simulink model "spi"  (Simulink 7.3)
settings: Solver=ode45  StartTime=0.0  StopTime=10.0  RelTol=1e-3
libraries: powerlib x11
settings Model: Creator=vlc  LastModifiedBy=vlc

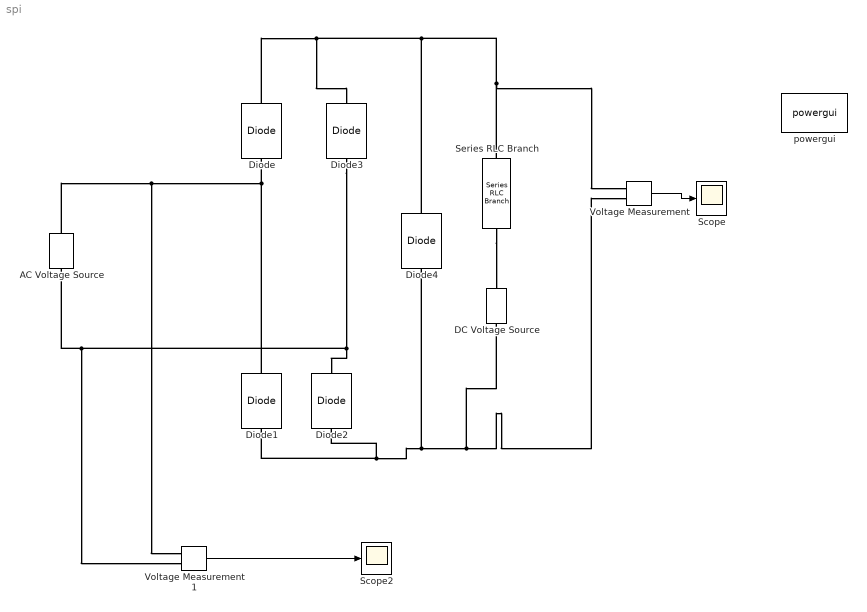
== system spi ==
  AC Voltage Source : powerlib/Electrical Sources/AC Voltage Source  DialogController=POWERSYS.PowerSysDialog  SystemSampleTime=-1  Amplitude=230  Phase=0  Frequency=50  SampleTime=0  Measurements=Voltage
  DC Voltage Source : powerlib/Electrical Sources/DC Voltage Source  DialogController=POWERSYS.PowerSysDialog  SystemSampleTime=-1  Amplitude=60  Measurements=None
  Diode : powerlib/Power Electronics/Diode  DialogController=POWERSYS.PowerSysDialog  SystemSampleTime=-1  Ron=.001  Lon=0  Vf=0.8  IC=0  UseSnubber=off  Rs=500  Cs=.0001  Measurements=off
  Diode1 : powerlib/Power Electronics/Diode  DialogController=POWERSYS.PowerSysDialog  SystemSampleTime=-1  Ron=0.001  Lon=0  Vf=0.8  IC=0  UseSnubber=off  Rs=500  Cs=.0001  Measurements=off
  Diode2 : powerlib/Power Electronics/Diode  DialogController=POWERSYS.PowerSysDialog  SystemSampleTime=-1  Ron=0.001  Lon=0  Vf=0.8  IC=0  UseSnubber=off  Rs=500  Cs=.0001  Measurements=off
  Diode3 : powerlib/Power Electronics/Diode  DialogController=POWERSYS.PowerSysDialog  SystemSampleTime=-1  Ron=0.001  Lon=0  Vf=0.8  IC=0  UseSnubber=off  Rs=500  Cs=0.0001  Measurements=off
  Diode4 : powerlib/Power Electronics/Diode  DialogController=POWERSYS.PowerSysDialog  SystemSampleTime=-1  Ron=0.001  Lon=0  Vf=0.8  IC=0  UseSnubber=off  Rs=500  Cs=0.0001  Measurements=off
  Scope : Scope
      settings: TickLabels=on  YMin=0.4923714759535655  YMax=0.8923714759535655
  Scope2 : Scope
      settings: SaveName=ScopeData2
  Series RLC Branch : powerlib/Elements/Series RLC Branch  DialogController=POWERSYS.PowerSysDialog  PhysicalDomain=powersysdomain  SubClassName=unknown  LeftPortType=p1  RightPortType=p1  LConnTagsString=__new0  RConnTagsString=__new0  BranchType=RL  Resistance=10  Inductance=.005  SetiL0=on  InitialCurrent=0  Capacitance=1.0  Setx0=off  InitialVoltage=0  Measurements=Branch voltage and current
  Voltage Measurement : powerlib/Measurements/Voltage Measurement  DialogController=POWERSYS.PowerSysDialog  SystemSampleTime=-1  PhasorSimulation=off  OutputType=Complex  PSBequivalent=0
  Voltage Measurement1 : powerlib/Measurements/Voltage Measurement  DialogController=POWERSYS.PowerSysDialog  SystemSampleTime=-1  PhasorSimulation=off  OutputType=Complex  PSBequivalent=0
  powergui : powerlib/powergui  Priority=1  SystemSampleTime=-1  SimulationMode=Discrete  SampleTime=50e-6  frequency=60  SPID=off  DisableSnubberDevices=on  DisableRonSwitches=off  DisableVfSwitches=off  SwTol=0  Interpol=off  frequencyindice=50  echomessages=off  HookPort=off  DisplayEquations=off  FunctionMessages=off  EnableUseOfTLC=off  x0status=steady  RestoreLinks=warning  Frange=[0:2:500]  Ylog=off  Xlog=on  ShowGrid=off  save=off  variable=ZData  ZoomFFT=on  StartTime=0.0  cycles=1  DisplayStyle=1  fundamental=60  FreqAxis=off  MaxFrequency=1000  frequencyindicesteady=1  RmsSteady=1  display=off  Ts=0  methode=off
  wires:
  Voltage Measurement1/1 -> Scope2/1
  Voltage Measurement/1 -> Scope/1
  connections:
  Voltage Measurement/LConn1 -- Series RLC Branch/LConn1 -- Diode/RConn1 -- Diode3/RConn1 -- Diode4/RConn1
  Diode1/LConn1 -- Diode2/LConn1 -- Voltage Measurement/LConn2 -- DC Voltage Source/LConn1 -- Diode4/LConn1
  AC Voltage Source/RConn1 -- Voltage Measurement1/LConn1 -- Diode/LConn1 -- Diode1/RConn1
  Diode3/LConn1 -- Diode2/RConn1 -- AC Voltage Source/LConn1 -- Voltage Measurement1/LConn2
  Series RLC Branch/RConn1 -- DC Voltage Source/RConn1
